simulink model "lighting"  (R2018b)
settings: Solver=VariableStepAuto  StartTime=0.0  StopTime=intervals  RelTol=1e-3
libraries: simulink x6
settings Model: Creator=Filipowicz_user1  LastModifiedBy=Filipowicz_user1

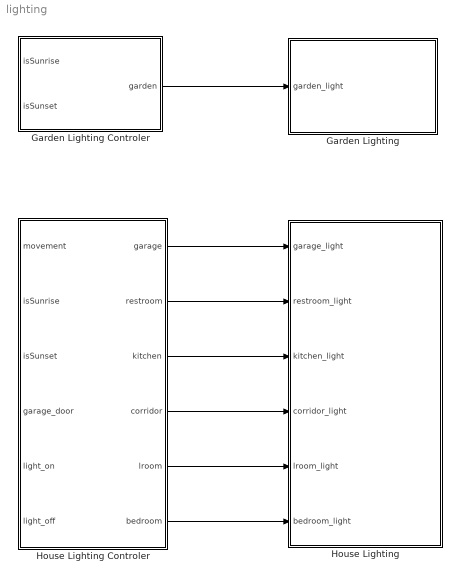
== system lighting ==
  Garden Lighting : Subsystem
  Garden Lighting Controler : Subsystem
  House Lighting : Subsystem
  House Lighting Controler : Subsystem
  wires:
  House Lighting Controler/1(garage) -> House Lighting/1(garage_light)
  House Lighting Controler/2(restroom) -> House Lighting/2(restroom_light)
  House Lighting Controler/3(kitchen) -> House Lighting/3(kitchen_light)
  House Lighting Controler/4(corridor) -> House Lighting/4(corridor_light)
  House Lighting Controler/5(lroom) -> House Lighting/5(lroom_light)
  House Lighting Controler/6(bedroom) -> House Lighting/6(bedroom_light)
  Garden Lighting Controler/1(garden) -> Garden Lighting/1(garden_light)

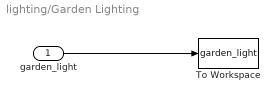
== system lighting/Garden Lighting ==
  garden_light : Inport
  To Workspace : ToWorkspace  VariableName=garden_light  SaveFormat=Timeseries  SampleTime=-1
  wires:
  garden_light/1 -> To Workspace/1

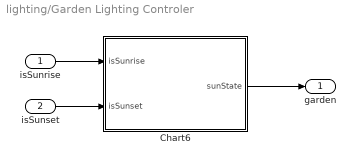
== system lighting/Garden Lighting Controler ==
  isSunrise : Inport
  isSunset : Inport  Port=2
  Chart6 : Stateflow chart  TreatAsAtomicUnit=on
  garden : Outport
  wires:
  isSunset/1 -> Chart6/2(isSunset)
  Chart6/1(sunState) -> garden/1
  isSunrise/1 -> Chart6/1(isSunrise)

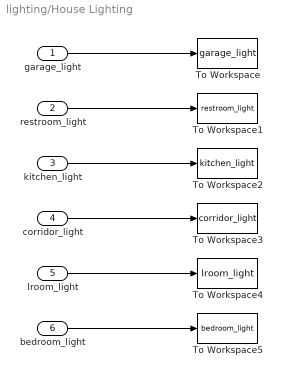
== system lighting/House Lighting ==
  garage_light : Inport
  restroom_light : Inport  Port=2
  kitchen_light : Inport  Port=3
  corridor_light : Inport  Port=4
  lroom_light : Inport  Port=5
  bedroom_light : Inport  Port=6
  To Workspace : ToWorkspace  VariableName=garage_light  SaveFormat=Timeseries  SampleTime=-1
  To Workspace1 : ToWorkspace  VariableName=restroom_light  SaveFormat=Timeseries  SampleTime=-1
  To Workspace2 : ToWorkspace  VariableName=kitchen_light  SaveFormat=Timeseries  SampleTime=-1
  To Workspace3 : ToWorkspace  VariableName=corridor_light  SaveFormat=Timeseries  SampleTime=-1
  To Workspace4 : ToWorkspace  VariableName=lroom_light  SaveFormat=Timeseries  SampleTime=-1
  To Workspace5 : ToWorkspace  VariableName=bedroom_light  SaveFormat=Timeseries  SampleTime=-1
  wires:
  kitchen_light/1 -> To Workspace2/1
  lroom_light/1 -> To Workspace4/1
  restroom_light/1 -> To Workspace1/1
  corridor_light/1 -> To Workspace3/1
  garage_light/1 -> To Workspace/1
  bedroom_light/1 -> To Workspace5/1

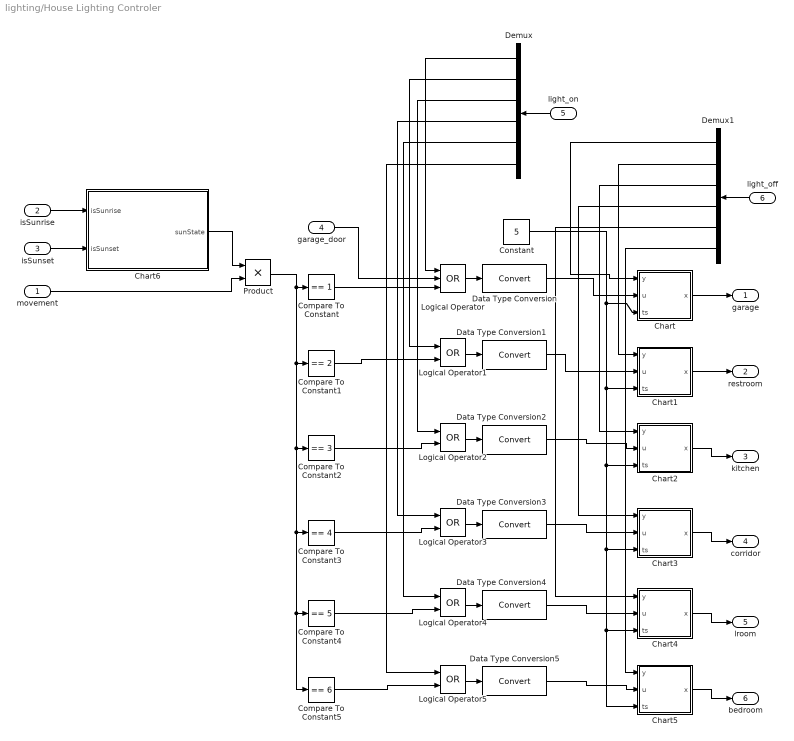
== system lighting/House Lighting Controler ==
  movement : Inport
  isSunrise : Inport  Port=2
  isSunset : Inport  Port=3
  garage_door : Inport  Port=4
  light_on : Inport  Port=5
  light_off : Inport  Port=6
  Chart : Stateflow chart  TreatAsAtomicUnit=on
  Chart1 : Stateflow chart  TreatAsAtomicUnit=on
  Chart2 : Stateflow chart  TreatAsAtomicUnit=on
  Chart3 : Stateflow chart  TreatAsAtomicUnit=on
  Chart4 : Stateflow chart  TreatAsAtomicUnit=on
  Chart5 : Stateflow chart  TreatAsAtomicUnit=on
  Chart6 : Stateflow chart  TreatAsAtomicUnit=on
  Compare To Constant : simulink/Logic and Bit Operations/Compare To Constant  relop===  const=1  OutDataTypeStr=boolean
  Compare To Constant1 : simulink/Logic and Bit Operations/Compare To Constant  relop===  const=2  OutDataTypeStr=boolean
  Compare To Constant2 : simulink/Logic and Bit Operations/Compare To Constant  relop===  const=3  OutDataTypeStr=boolean
  Compare To Constant3 : simulink/Logic and Bit Operations/Compare To Constant  relop===  const=4  OutDataTypeStr=boolean
  Compare To Constant4 : simulink/Logic and Bit Operations/Compare To Constant  relop===  const=5  OutDataTypeStr=boolean
  Compare To Constant5 : simulink/Logic and Bit Operations/Compare To Constant  relop===  const=6  OutDataTypeStr=boolean
  Constant : Constant  Value=5
  Data Type Conversion{,1..5} (6 alike) : DataTypeConversion
  Demux : Demux  Outputs=6
  Demux1 : Demux  Outputs=6
  Logical Operator : Logic  Operator=OR  Inputs=3  AllPortsSameDT=off  OutDataTypeStr=boolean
  Logical Operator{1..5} (5 alike) : Logic  Operator=OR  AllPortsSameDT=off  OutDataTypeStr=boolean
  Product : Product
  garage : Outport
  restroom : Outport  Port=2
  kitchen : Outport  Port=3
  corridor : Outport  Port=4
  lroom : Outport  Port=5
  bedroom : Outport  Port=6
  wires:
  movement/1 -> Product/2
  Constant/1 -> Chart/3(ts), Chart1/3(ts), Chart2/3(ts), Chart3/3(ts), Chart5/3(ts), Chart4/3(ts)
  Data Type Conversion/1 -> Chart/2(u)
  Data Type Conversion1/1 -> Chart1/2(u)
  Data Type Conversion2/1 -> Chart2/2(u)
  Data Type Conversion3/1 -> Chart3/2(u)
  Data Type Conversion4/1 -> Chart4/2(u)
  Data Type Conversion5/1 -> Chart5/2(u)
  isSunset/1 -> Chart6/2(isSunset)
  isSunrise/1 -> Chart6/1(isSunrise)
  Chart6/1(sunState) -> Product/1
  Product/1 -> Compare To Constant5/1, Compare To Constant4/1, Compare To Constant3/1, Compare To Constant2/1, Compare To Constant1/1, Compare To Constant/1
  Compare To Constant/1 -> Logical Operator/3
  Logical Operator/1 -> Data Type Conversion/1
  garage_door/1 -> Logical Operator/2
  Chart/1(x) -> garage/1
  Chart1/1(x) -> restroom/1
  Chart2/1(x) -> kitchen/1
  Chart3/1(x) -> corridor/1
  Chart4/1(x) -> lroom/1
  Chart5/1(x) -> bedroom/1
  Demux/1 -> Logical Operator/1
  Logical Operator1/1 -> Data Type Conversion1/1
  Compare To Constant1/1 -> Logical Operator1/2
  Demux/2 -> Logical Operator1/1
  Logical Operator2/1 -> Data Type Conversion2/1
  Logical Operator3/1 -> Data Type Conversion3/1
  Logical Operator4/1 -> Data Type Conversion4/1
  Logical Operator5/1 -> Data Type Conversion5/1
  Demux/3 -> Logical Operator2/1
  Demux/4 -> Logical Operator3/1
  Demux/5 -> Logical Operator4/1
  Demux/6 -> Logical Operator5/1
  Compare To Constant2/1 -> Logical Operator2/2
  Compare To Constant3/1 -> Logical Operator3/2
  Compare To Constant4/1 -> Logical Operator4/2
  Compare To Constant5/1 -> Logical Operator5/2
  light_on/1 -> Demux/1
  Demux1/1 -> Chart/1(y)
  Demux1/2 -> Chart1/1(y)
  Demux1/3 -> Chart2/1(y)
  Demux1/4 -> Chart3/1(y)
  Demux1/5 -> Chart4/1(y)
  Demux1/6 -> Chart5/1(y)
  light_off/1 -> Demux1/1

== stateflow chart lighting/House Lighting Controler/Chart1 ==
  settings: updateMethod=DISCRETE  sampleTime=1  executeAtInitialization=1
  state Idle
    x=0;
    t1=ts/timeStep;
  state State1
    x=1;
  state Wait
  (default) -> Idle
  Idle -> Idle [order 2]
  Wait -> Idle [order 2] : after(t1,'sec')
  Idle -> State1 [order 1] : [u>=1]
  State1 -> Idle [order 2] : [y==1]
  State1 -> Wait [order 1] : [u==0]
  Wait -> State1 [order 1] : [u==1]
  data: y input; u input; x output; ts input; timeStep constant double; t1 local

== stateflow chart lighting/House Lighting Controler/Chart2 ==
  settings: updateMethod=DISCRETE  sampleTime=1  executeAtInitialization=1
  state Idle
    x=0;
    t1=ts/timeStep;
  state State1
    x=1;
  state Wait
  (default) -> Idle
  Idle -> Idle [order 2]
  Wait -> Idle [order 2] : after(t1,'sec')
  Idle -> State1 [order 1] : [u>=1]
  State1 -> Idle [order 2] : [y==1]
  State1 -> Wait [order 1] : [u==0]
  Wait -> State1 [order 1] : [u==1]
  data: y input; u input; x output; ts input; timeStep constant double; t1 local

== stateflow chart lighting/House Lighting Controler/Chart ==
  settings: updateMethod=DISCRETE  sampleTime=1  executeAtInitialization=1
  state Idle
    x=0;
    t1=ts/timeStep;
  state State1
    x=1;
  state Wait
  (default) -> Idle
  Idle -> Idle [order 2]
  Wait -> Idle [order 2] : after(t1,'sec')
  Idle -> State1 [order 1] : [u>=1]
  State1 -> Idle [order 2] : [y==1]
  State1 -> Wait [order 1] : [u==0]
  Wait -> State1 [order 1] : [u==1]
  data: y input; u input; x output; ts input; timeStep constant double; t1 local

== stateflow chart lighting/House Lighting Controler/Chart3 ==
  settings: updateMethod=DISCRETE  sampleTime=1  executeAtInitialization=1
  state Idle
    x=0;
    t1=ts/timeStep;
  state State1
    x=1;
  state Wait
  (default) -> Idle
  Idle -> Idle [order 2]
  Wait -> Idle [order 2] : after(t1,'sec')
  Idle -> State1 [order 1] : [u>=1]
  State1 -> Idle [order 2] : [y==1]
  State1 -> Wait [order 1] : [u==0]
  Wait -> State1 [order 1] : [u==1]
  data: y input; u input; x output; ts input; timeStep constant double; t1 local

== stateflow chart lighting/House Lighting Controler/Chart4 ==
  settings: updateMethod=DISCRETE  sampleTime=1  executeAtInitialization=1
  state Idle
    x=0;
    t1=ts/timeStep;
  state State1
    x=1;
  state Wait
  (default) -> Idle
  Idle -> Idle [order 2]
  Wait -> Idle [order 2] : after(t1,'sec')
  Idle -> State1 [order 1] : [u>=1]
  State1 -> Idle [order 2] : [y==1]
  State1 -> Wait [order 1] : [u==0]
  Wait -> State1 [order 1] : [u==1]
  data: y input; u input; x output; ts input; timeStep constant double; t1 local

== stateflow chart lighting/House Lighting Controler/Chart5 ==
  settings: updateMethod=DISCRETE  sampleTime=1  executeAtInitialization=1
  state Idle
    x=0;
    t1=ts/timeStep;
  state State1
    x=1;
  state Wait
  (default) -> Idle
  Idle -> Idle [order 2]
  Wait -> Idle [order 2] : after(t1,'sec')
  Idle -> State1 [order 1] : [u>=1]
  State1 -> Idle [order 2] : [y==1]
  State1 -> Wait [order 1] : [u==0]
  Wait -> State1 [order 1] : [u==1]
  data: y input; u input; x output; ts input; timeStep constant double; t1 local

== stateflow chart lighting/House Lighting Controler/Chart6 ==
  settings: updateMethod=DISCRETE  sampleTime=1  executeAtInitialization=1
  state sun_up
    sunState=0;
  state sun_down
    sunState=1;
  (default) -> sun_up
  sun_up -> sun_down : [isSunrise]
  sun_down -> sun_up : [isSunset]
  data: isSunrise input; isSunset input; sunState output

== stateflow chart lighting/Garden Lighting Controler/Chart6 ==
  settings: updateMethod=DISCRETE  sampleTime=1  executeAtInitialization=1
  state sun_up
    sunState=0;
  state sun_down
    sunState=1;
  (default) -> sun_up
  sun_up -> sun_down : [isSunrise]
  sun_down -> sun_up : [isSunset]
  data: isSunrise input; isSunset input; sunState output
